simulink model "observer"  (R2018a)
settings: Solver=VariableStepAuto  StartTime=0.0  StopTime=10.0  RelTol=1e-3
values from neighbouring files (symbols this model uses):
  a = [-20.6 0; 0 -1]    [start.m]
  b = [0 1]'    [start.m]
  ce = [1 ,1]    [start.m]
  L = L_T'    [start.m]
settings Model: Creator=maroufi  LastModifiedBy=maroufi

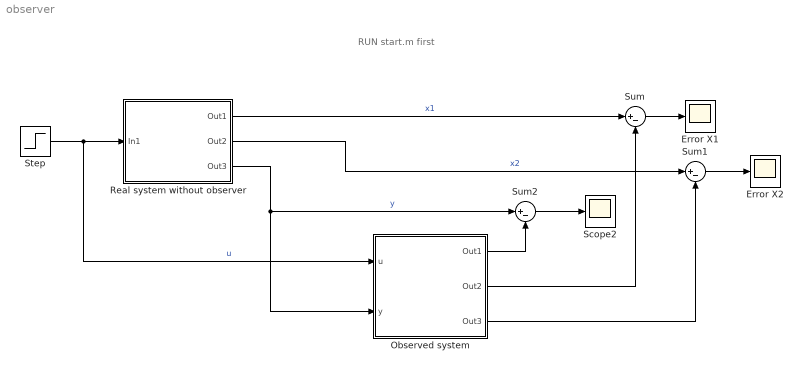
== system observer ==
  note: RUN start.m first
  Error X1 : Scope
  Error X2 : Scope
  Observed system : Subsystem
  Real system without observer : Subsystem
  Scope2 : Scope
  Step : Step  SampleTime=0
  Sum : Sum  Inputs=|+-
  Sum1 : Sum  Inputs=|+-
  Sum2 : Sum  Inputs=|+-
  wires:
  Step/1 -> Observed system/1(u), Real system without observer/1(In1)  "u"
  Real system without observer/1(Out1) -> Sum/1  "x1"
  Real system without observer/2(Out2) -> Sum1/1  "x2"
  Real system without observer/3(Out3) -> Sum2/1, Observed system/2(y)  "y"
  Observed system/2(Out2) -> Sum/2
  Observed system/3(Out3) -> Sum1/2
  Observed system/1(Out1) -> Sum2/2
  Sum/1 -> Error X1/1
  Sum1/1 -> Error X2/1
  Sum2/1 -> Scope2/1

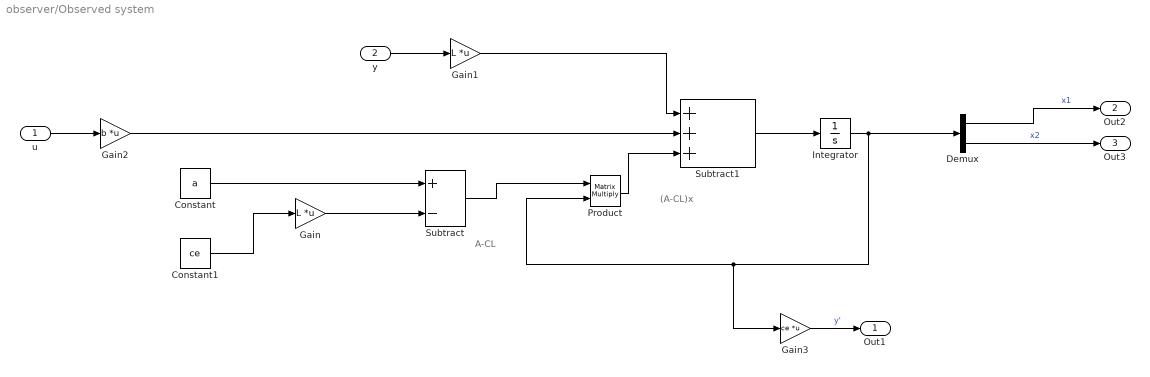
== system observer/Observed system ==
  note: A-CL
  note: (A-CL)x
  u : Inport
  y : Inport  Port=2
  Constant : Constant  Value=a
  Constant1 : Constant  Value=ce  VectorParams1D=off
  Demux : Demux  Outputs=2
  Gain : Gain  Gain=L  Multiplication=Matrix(K*u)
  Gain1 : Gain  Gain=L  Multiplication=Matrix(K*u)
  Gain2 : Gain  Gain=b  Multiplication=Matrix(K*u)
  Gain3 : Gain  Gain=ce  Multiplication=Matrix(K*u)
  Integrator : Integrator
  Product : Product  Multiplication=Matrix(*)
  Subtract : Sum  Inputs=+-
  Subtract1 : Sum  Inputs=+++
  Out1 : Outport
  Out2 : Outport  Port=2
  Out3 : Outport  Port=3
  wires:
  Integrator/1 -> Demux/1, Product/2, Gain3/1
  Subtract1/1 -> Integrator/1
  Gain2/1 -> Subtract1/2
  u/1 -> Gain2/1
  y/1 -> Gain1/1
  Gain/1 -> Subtract/2
  Product/1 -> Subtract1/3
  Constant/1 -> Subtract/1
  Gain1/1 -> Subtract1/1
  Gain3/1 -> Out1/1  "y'"
  Demux/1 -> Out2/1  "x1"
  Demux/2 -> Out3/1  "x2"
  Constant1/1 -> Gain/1
  Subtract/1 -> Product/1

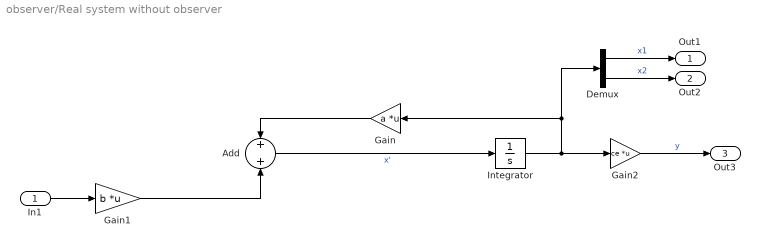
== system observer/Real system without observer ==
  In1 : Inport
  Add : Sum
  Demux : Demux  Outputs=2
  Gain : Gain  Gain=a  Multiplication=Matrix(K*u)
  Gain1 : Gain  Gain=b  Multiplication=Matrix(K*u)
  Gain2 : Gain  Gain=ce  Multiplication=Matrix(K*u)
  Integrator : Integrator  InitialCondition=[1,1]
  Out1 : Outport
  Out2 : Outport  Port=2
  Out3 : Outport  Port=3
  wires:
  Gain/1 -> Add/1
  Gain1/1 -> Add/2
  Add/1 -> Integrator/1  "x'"
  Demux/1 -> Out1/1  "x1"
  In1/1 -> Gain1/1
  Integrator/1 -> Gain2/1, Demux/1, Gain/1
  Demux/2 -> Out2/1  "x2"
  Gain2/1 -> Out3/1  "y"
